simulink model "exp3"  (R2024a)
settings: Solver=VariableStepAuto  StartTime=0.0  StopTime=10.0  RelTol=1e-3
libraries: dspsrcs4 x5, simulink x4
settings RTWCC: GPUComputeCapability=3.5

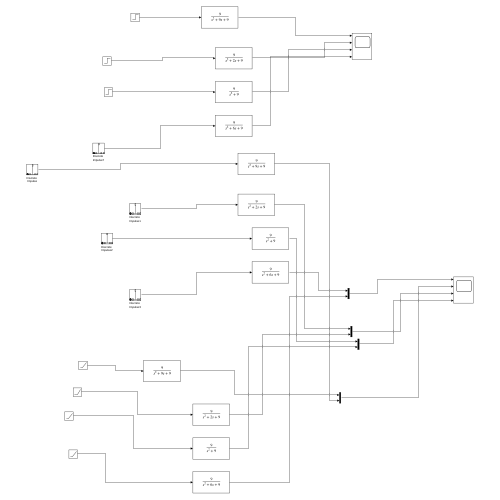
[thumbnail: Simulink's stored preview of the top-level diagram]
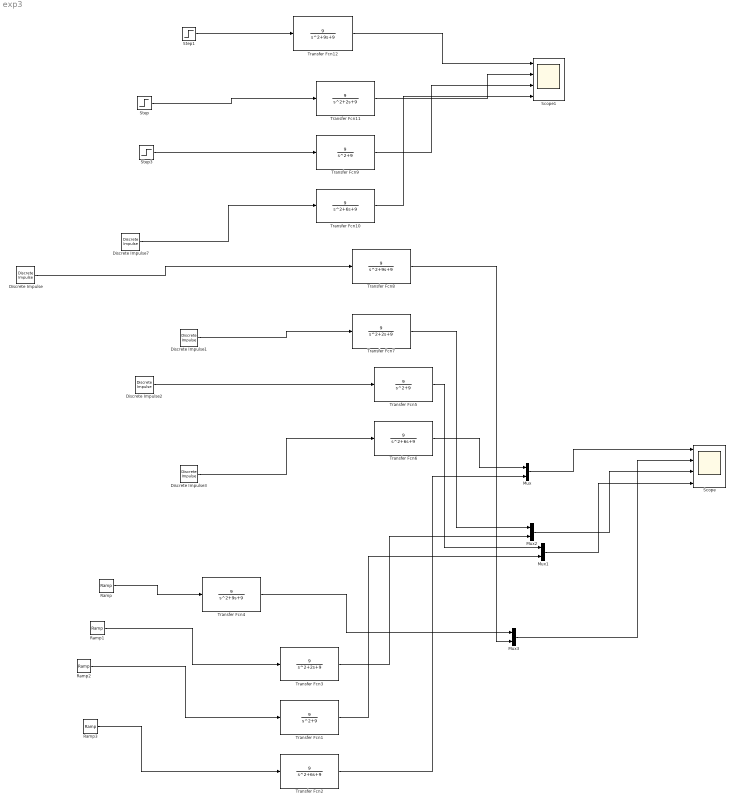
== system exp3 ==
  Discrete Impulse{,1..3,7} (5 alike) : dspsrcs4/Discrete  Impulse  Delay=0  SampleTime=1  FrameSample=1  OutputFrames=off  dataType=double  isSigned=on  wordLen=16  udDataType=sfix(16)  fracBitsMode=Best precision  numFracBits=15  OutDataTypeStr=double  LastOutDataTypeStr=double
  Mux{,1..3} (4 alike) : Mux  Inputs=2
  Ramp{,1..3} (4 alike) : simulink/Sources/Ramp  slope=1  start=0  InitialOutput=0
  Scope : Scope  NumInputPorts=4
  Scope1 : Scope  NumInputPorts=4
  Step : Step  SampleTime=0
  Step1 : Step  SampleTime=0
  Step3 : Step  SampleTime=0
  Transfer Fcn1 : TransferFcn  Numerator=[9]  Denominator=[1 0 9]
  Transfer Fcn10 : TransferFcn  Numerator=[9]  Denominator=[1 6 9]
  Transfer Fcn11 : TransferFcn  Numerator=[9]  Denominator=[1 2 9]
  Transfer Fcn12 : TransferFcn  Numerator=[9]  Denominator=[1 9 9]
  Transfer Fcn2 : TransferFcn  Numerator=[9]  Denominator=[1 6 9]
  Transfer Fcn3 : TransferFcn  Numerator=[9]  Denominator=[1 2 9]
  Transfer Fcn4 : TransferFcn  Numerator=[9]  Denominator=[1 9 9]
  Transfer Fcn5 : TransferFcn  Numerator=[9]  Denominator=[1 0 9]
  Transfer Fcn6 : TransferFcn  Numerator=[9]  Denominator=[1 6 9]
  Transfer Fcn7 : TransferFcn  Numerator=[9]  Denominator=[1 2 9]
  Transfer Fcn8 : TransferFcn  Numerator=[9]  Denominator=[1 9 9]
  Transfer Fcn9 : TransferFcn  Numerator=[9]  Denominator=[1 0 9]
  wires:
  Ramp/1 -> Transfer Fcn4/1
  Ramp1/1 -> Transfer Fcn3/1
  Ramp2/1 -> Transfer Fcn1/1
  Ramp3/1 -> Transfer Fcn2/1
  Discrete Impulse3/1 -> Transfer Fcn6/1
  Discrete Impulse2/1 -> Transfer Fcn5/1
  Discrete Impulse/1 -> Transfer Fcn8/1
  Discrete Impulse1/1 -> Transfer Fcn7/1
  Transfer Fcn6/1 -> Mux/1
  Transfer Fcn2/1 -> Mux/2
  Mux/1 -> Scope/1
  Transfer Fcn4/1 -> Mux3/1
  Transfer Fcn8/1 -> Mux3/2
  Mux3/1 -> Scope/2
  Transfer Fcn7/1 -> Mux2/1
  Mux2/1 -> Scope/3
  Transfer Fcn3/1 -> Mux2/2
  Transfer Fcn1/1 -> Mux1/2
  Transfer Fcn5/1 -> Mux1/1
  Mux1/1 -> Scope/4
  Discrete Impulse7/1 -> Transfer Fcn10/1
  Step3/1 -> Transfer Fcn9/1
  Step1/1 -> Transfer Fcn12/1
  Step/1 -> Transfer Fcn11/1
  Transfer Fcn12/1 -> Scope1/1
  Transfer Fcn11/1 -> Scope1/2
  Transfer Fcn9/1 -> Scope1/3
  Transfer Fcn10/1 -> Scope1/4
